simulink model "PlantLinearizer"  (R2016a)
settings: Solver=VariableStepAuto  StartTime=0.0  StopTime=10.0  RelTol=1e-3
libraries: SimMainLibrary x1
settings Model: Creator=dtk42  LastModifiedBy=dtk42

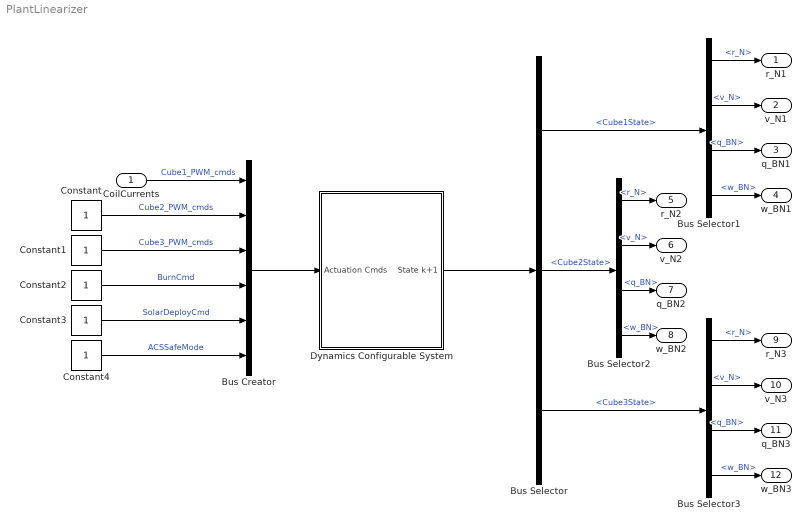
== system PlantLinearizer ==
  CoilCurrents : Inport
  Bus Creator : BusCreator  Inputs=6
  Bus Selector : BusSelector  OutputSignals=Cube1State,Cube2State,Cube3State
  Bus Selector1 : BusSelector  OutputSignals=r_N,v_N,q_BN,w_BN
  Bus Selector2 : BusSelector  OutputSignals=r_N,v_N,q_BN,w_BN
  Bus Selector3 : BusSelector  OutputSignals=r_N,v_N,q_BN,w_BN
  Constant{,1..4} (5 alike) : Constant
  Dynamics Configurable System : Subsystem  BlockChoice=Simscape 1 Piece Tether
      settings: AttributesFormatString=%<BlockChoice>  TemplateBlock=SimMainLibrary/Dynamics Configurable System  MemberBlocks=Dynamics By Hand,Simscape 1 Piece Tether,Simscape 3 Piece Tether
  r_N1 : Outport
  v_N1 : Outport  Port=2
  q_BN1 : Outport  Port=3
  w_BN1 : Outport  Port=4
  r_N2 : Outport  Port=5
  v_N2 : Outport  Port=6
  q_BN2 : Outport  Port=7
  w_BN2 : Outport  Port=8
  r_N3 : Outport  Port=9
  v_N3 : Outport  Port=10
  q_BN3 : Outport  Port=11
  w_BN3 : Outport  Port=12
  wires:
  Dynamics Configurable System/1(State k+1) -> Bus Selector/1
  Bus Selector/1 -> Bus Selector1/1  "<Cube1State>"
  Bus Selector/2 -> Bus Selector2/1  "<Cube2State>"
  Bus Selector/3 -> Bus Selector3/1  "<Cube3State>"
  Bus Selector1/1 -> r_N1/1  "<r_N>"
  Bus Selector1/2 -> v_N1/1  "<v_N>"
  Bus Selector1/3 -> q_BN1/1  "<q_BN>"
  Bus Selector1/4 -> w_BN1/1  "<w_BN>"
  Bus Selector2/1 -> r_N2/1  "<r_N>"
  Bus Selector2/2 -> v_N2/1  "<v_N>"
  Bus Selector2/3 -> q_BN2/1  "<q_BN>"
  Bus Selector2/4 -> w_BN2/1  "<w_BN>"
  Bus Selector3/1 -> r_N3/1  "<r_N>"
  Bus Selector3/2 -> v_N3/1  "<v_N>"
  Bus Selector3/3 -> q_BN3/1  "<q_BN>"
  Bus Selector3/4 -> w_BN3/1  "<w_BN>"
  Bus Creator/1 -> Dynamics Configurable System/1(Actuation Cmds)
  CoilCurrents/1 -> Bus Creator/1  "Cube1_PWM_cmds"
  Constant/1 -> Bus Creator/2  "Cube2_PWM_cmds"
  Constant1/1 -> Bus Creator/3  "Cube3_PWM_cmds"
  Constant2/1 -> Bus Creator/4  "BurnCmd"
  Constant3/1 -> Bus Creator/5  "SolarDeployCmd"
  Constant4/1 -> Bus Creator/6  "ACSSafeMode"

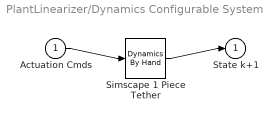
== system PlantLinearizer/Dynamics Configurable System ==
  Actuation Cmds : Inport
  Simscape 1 Piece Tether : SimMainLibrary/Dynamics By Hand
  State k+1 : Outport
  wires:
  Actuation Cmds/1 -> Simscape 1 Piece Tether/1
  Simscape 1 Piece Tether/1 -> State k+1/1
